simulink model "cdma_1"  (Simulink 7.8)
settings: Solver=ode45  StartTime=0.0  StopTime=10.0  RelTol=1e-3
undefined symbols (not defined in the file or in its folder): Fs, get, sided, Two
libraries: commrandsrc2 x10, commseqgen2 x10, commsink2 x3, dsparch4 x3, commutil2 x2, commdigbbndpm3 x2, dspsnks4 x2, commchan3 x1
settings Model: Creator=Administrator  LastModifiedBy=Administrator

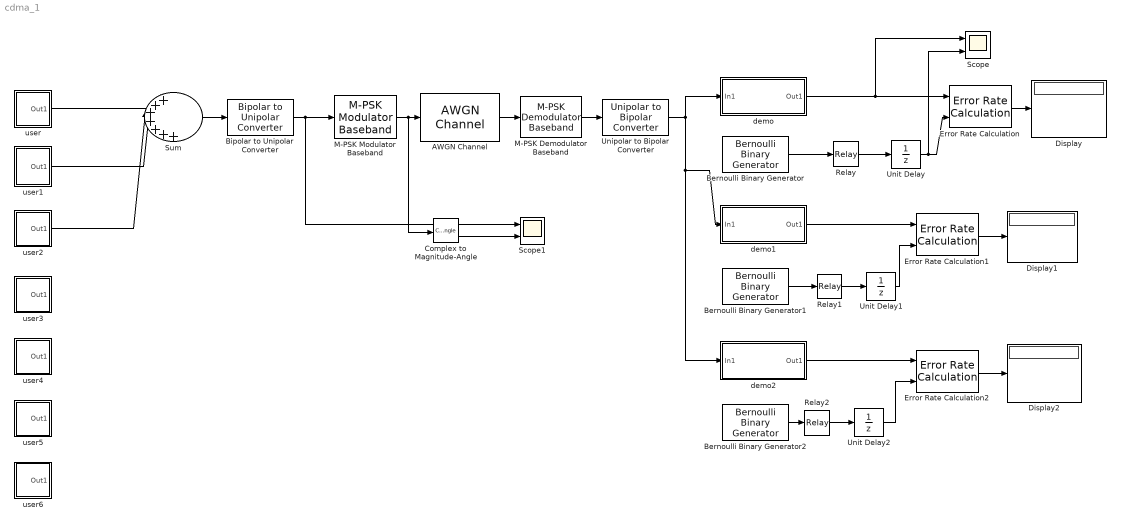
== system cdma_1 ==
  AWGN Channel : commchan3/AWGN Channel  InputProcessing=Columns as channels (frame based)  seed=1567  noiseMode="Signal to noise ratio  (SNR)"  EbNodB=10  EsNodB=10  SNRdB=10  bitsPerSym=1  Ps=1  Tsym=1  variance=1
  Bernoulli Binary Generator : commrandsrc2/Bernoulli Binary Generator  P=0.5  seed=67  Ts=6e-4  frameBased=off  sampPerFrame=1  orient=off  outDataType=double
  Bernoulli Binary Generator1 : commrandsrc2/Bernoulli Binary Generator  P=0.5  seed=71  Ts=6e-4  frameBased=off  sampPerFrame=1  orient=off  outDataType=double
  Bernoulli Binary Generator2 : commrandsrc2/Bernoulli Binary Generator  P=0.5  seed=87  Ts=6e-4  frameBased=off  sampPerFrame=1  orient=off  outDataType=double
  Bipolar to Unipolar Converter : commutil2/Bipolar to Unipolar Converter  M=4  polarity=Positive  dataType=Inherit via internal rule
  Complex to Magnitude-Angle : ComplexToMagnitudeAngle
  Display : Display
  Display1 : Display
  Display2 : Display
  Error Rate Calculation : commsink2/Error Rate Calculation  N=0  st_delay=0  cp_mode=Entire frame  subframe=[]  PMode=Port  WsName=ErrorVec  RsMode2=off  stop=off  numErr=100  maxBits=1e6
  Error Rate Calculation1 : commsink2/Error Rate Calculation  N=0  st_delay=0  cp_mode=Entire frame  subframe=[]  PMode=Port  WsName=ErrorVec  RsMode2=off  stop=off  numErr=100  maxBits=1e6
  Error Rate Calculation2 : commsink2/Error Rate Calculation  N=0  st_delay=0  cp_mode=Entire frame  subframe=[]  PMode=Port  WsName=ErrorVec  RsMode2=off  stop=off  numErr=100  maxBits=1e6
  M-PSK Demodulator Baseband : commdigbbndpm3/M-PSK Demodulator Baseband  M=4  Ph=pi/4  Dec=Gray  Mapping=[0:7]  OutType=Integer  DecType=Hard decision  VarSource=Dialog  Variance=1  outDtype1=Inherit via internal rule  outDtype2=Inherit via internal rule  derotateFactorWordLen=16
  M-PSK Modulator Baseband : commdigbbndpm3/M-PSK Modulator Baseband  M=4  InType=Integer  Enc=Gray  Mapping=[0:7]  Ph=pi/4  outDtype=double  outWordLen=16  outUDDataType=sfix(16)  outFracLenMode=Best precision  outFracLen=15
  Relay : Relay  OnSwitchValue=0.9  OffSwitchValue=0.1  OffOutputValue=-1
  Relay1 : Relay  OnSwitchValue=0.9  OffSwitchValue=0.1  OffOutputValue=-1
  Relay2 : Relay  OnSwitchValue=0.9  OffSwitchValue=0.1  OffOutputValue=-1
  Scope : Scope  NumInputPorts=2
      settings: YMin=-2~-2  YMax=2~2
  Scope1 : Scope  NumInputPorts=2
      settings: YMin=1~-2  YMax=6~4  SaveName=ScopeData2
  Sum : Sum  Inputs=|+++++++
  Unipolar to Bipolar Converter : commutil2/Unipolar to Bipolar Converter  M=4  polarity=Positive  dataType=Inherit via internal rule
  Unit Delay : UnitDelay  SampleTime=-1
  Unit Delay1 : UnitDelay  SampleTime=-1
  Unit Delay2 : UnitDelay  SampleTime=-1
  demo : Subsystem
  demo1 : Subsystem
  demo2 : Subsystem
  user : Subsystem
  user1 : Subsystem
  user2 : Subsystem
  user3 : Subsystem
  user4 : Subsystem
  user5 : Subsystem
  user6 : Subsystem
  wires:
  Error Rate Calculation/1 -> Display/1
  Bernoulli Binary Generator/1 -> Relay/1
  Relay/1 -> Unit Delay/1
  Relay1/1 -> Unit Delay1/1
  Bernoulli Binary Generator1/1 -> Relay1/1
  AWGN Channel/1 -> M-PSK Demodulator Baseband/1
  user1/1(Out1) -> Sum/2
  user/1(Out1) -> Sum/1
  M-PSK Modulator Baseband/1 -> AWGN Channel/1, Complex to Magnitude-Angle/1
  M-PSK Demodulator Baseband/1 -> Unipolar to Bipolar Converter/1
  Bipolar to Unipolar Converter/1 -> M-PSK Modulator Baseband/1, Scope1/1
  Unipolar to Bipolar Converter/1 -> demo/1(In1), demo1/1(In1), demo2/1(In1)
  demo1/1(Out1) -> Error Rate Calculation1/1
  Bernoulli Binary Generator2/1 -> Relay2/1
  Relay2/1 -> Unit Delay2/1
  Error Rate Calculation1/1 -> Display1/1
  demo2/1(Out1) -> Error Rate Calculation2/1
  Error Rate Calculation2/1 -> Display2/1
  Unit Delay1/1 -> Error Rate Calculation1/2
  Unit Delay/1 -> Error Rate Calculation/2, Scope/2
  demo/1(Out1) -> Error Rate Calculation/1, Scope/1
  Unit Delay2/1 -> Error Rate Calculation2/2
  Sum/1 -> Bipolar to Unipolar Converter/1
  Complex to Magnitude-Angle/2 -> Scope1/2
  user2/1(Out1) -> Sum/3

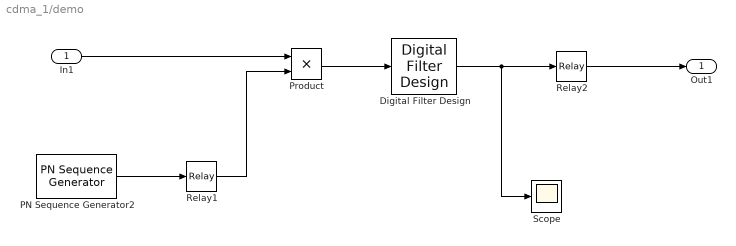
== system cdma_1/demo ==
  In1 : Inport
  Digital Filter Design : dsparch4/Digital Filter Design  mwdsp_browser_bugfix_var=off
  PN Sequence Generator2 : commseqgen2/PN Sequence Generator  poly=[1 0 0 0 0 1 1]  ini_sta=[0 0 0 0 0 1]  outBitMaskSource=Dialog parameter  shift=0  outVarSiz=off  maxOutSizeMode=Dialog parameter  maxOutSize=[10 1]  Ts=2e-5  frameBased=off  sampPerFrame=1  reset=off  bitPackedOutputs=off  outDataType=double  numPackedBits=8  bitPackDataSigned=off  bitPackedOutDType=double
  Product : Product  RndMeth=Zero
  Relay1 : Relay  OnSwitchValue=0.9  OffSwitchValue=0.1  OffOutputValue=-1
  Relay2 : Relay  OnSwitchValue=0  OffSwitchValue=0  OffOutputValue=-1  SampleTime=6e-4
  Scope : Scope
  Out1 : Outport
  wires:
  PN Sequence Generator2/1 -> Relay1/1
  Relay1/1 -> Product/2
  Relay2/1 -> Out1/1
  In1/1 -> Product/1
  Product/1 -> Digital Filter Design/1
  Digital Filter Design/1 -> Relay2/1, Scope/1

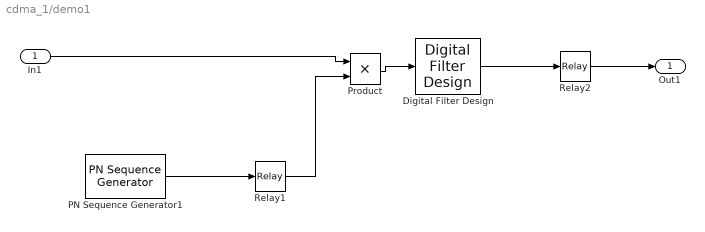
== system cdma_1/demo1 ==
  In1 : Inport
  Digital Filter Design : dsparch4/Digital Filter Design  mwdsp_browser_bugfix_var=off
  PN Sequence Generator1 : commseqgen2/PN Sequence Generator  poly=[1 0 0 0 0 1 1]  ini_sta=[1 0 0 0 0 0]  outBitMaskSource=Dialog parameter  shift=0  outVarSiz=off  maxOutSizeMode=Dialog parameter  maxOutSize=[10 1]  Ts=2e-5  frameBased=off  sampPerFrame=1  reset=off  bitPackedOutputs=off  outDataType=double  numPackedBits=8  bitPackDataSigned=off  bitPackedOutDType=double
  Product : Product  RndMeth=Zero
  Relay1 : Relay  OnSwitchValue=0.9  OffSwitchValue=0.1  OffOutputValue=-1
  Relay2 : Relay  OnSwitchValue=0  OffSwitchValue=0  OffOutputValue=-1  SampleTime=6e-4
  Out1 : Outport
  wires:
  Digital Filter Design/1 -> Relay2/1
  Relay1/1 -> Product/2
  Product/1 -> Digital Filter Design/1
  Relay2/1 -> Out1/1
  In1/1 -> Product/1
  PN Sequence Generator1/1 -> Relay1/1

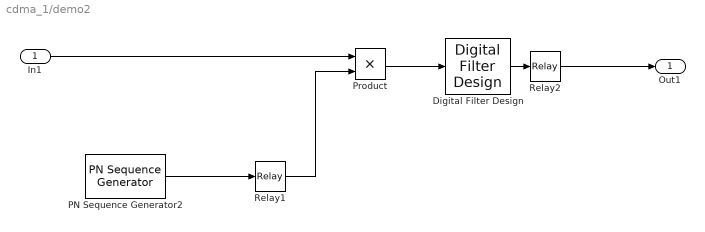
== system cdma_1/demo2 ==
  In1 : Inport
  Digital Filter Design : dsparch4/Digital Filter Design  mwdsp_browser_bugfix_var=off
  PN Sequence Generator2 : commseqgen2/PN Sequence Generator  poly=[1 0 0 0 0 1 1]  ini_sta=[1 1 0 0 0 0]  outBitMaskSource=Dialog parameter  shift=0  outVarSiz=off  maxOutSizeMode=Dialog parameter  maxOutSize=[10 1]  Ts=2e-5  frameBased=off  sampPerFrame=1  reset=off  bitPackedOutputs=off  outDataType=double  numPackedBits=8  bitPackDataSigned=off  bitPackedOutDType=double
  Product : Product  RndMeth=Zero
  Relay1 : Relay  OnSwitchValue=0.9  OffSwitchValue=0.1  OffOutputValue=-1
  Relay2 : Relay  OnSwitchValue=0  OffSwitchValue=0  OffOutputValue=-1  SampleTime=6e-4
  Out1 : Outport
  wires:
  Digital Filter Design/1 -> Relay2/1
  Relay1/1 -> Product/2
  Product/1 -> Digital Filter Design/1
  Relay2/1 -> Out1/1
  In1/1 -> Product/1
  PN Sequence Generator2/1 -> Relay1/1

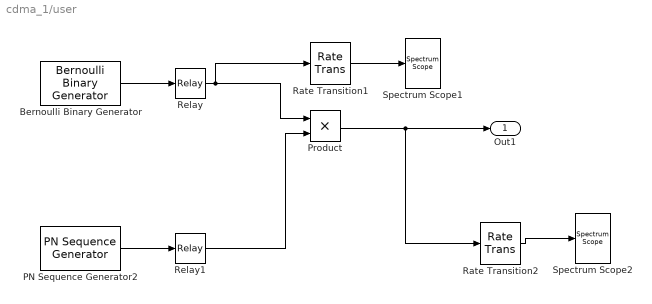
== system cdma_1/user ==
  Bernoulli Binary Generator : commrandsrc2/Bernoulli Binary Generator  P=0.5  seed=67  Ts=6e-4  frameBased=off  sampPerFrame=1  orient=off  outDataType=double
  PN Sequence Generator2 : commseqgen2/PN Sequence Generator  poly=[1 0 0 0 0 1 1]  ini_sta=[0 0 0 0 0 1]  outBitMaskSource=Dialog parameter  shift=0  outVarSiz=off  maxOutSizeMode=Dialog parameter  maxOutSize=[10 1]  Ts=2e-5  frameBased=off  sampPerFrame=1  reset=off  bitPackedOutputs=off  outDataType=double  numPackedBits=8  bitPackDataSigned=off  bitPackedOutDType=double
  Product : Product  RndMeth=Zero
  Rate Transition1 : RateTransition  OutPortSampleTime=1/10000
  Rate Transition2 : RateTransition  OutPortSampleTime=2/1000000
  Relay : Relay  OnSwitchValue=0.9  OffSwitchValue=0.1  OffOutputValue=-1
  Relay1 : Relay  OnSwitchValue=0.9  OffSwitchValue=0.1  OffOutputValue=-1
  Spectrum Scope1 : dspsnks4/Spectrum Scope  ScopeProperties=on  Domain=Frequency  HorizSpan=1  UseBuffer=on  BufferSize=2048  Overlap=0  TreatMby1Signals=One channel  inpFftLenInherit=off  FFTlength=128  numAvg=2  DisplayProperties=off  AxisGrid=on  Memory=off  FrameNumber=on  AxisLegend=off  AxisZoom=off  OpenScopeAtSimStart=on  OpenScopeImmediately=off  FigPos=get(0,'defaultfigureposition')  AxisProperties=off  XUnits=Hertz  XRange=Two-sided ((-Fs/2...Fs/2])  XDisplay=0  InheritXIncr=on  XIncr=1.0  XLabel=Samples  XLimit=Auto  YUnits=dBm  XMax=1  XMin=0  YLabel=Magnitude-squared, dB  LineProperties=off  wintypeSpecScope=Hann  RsSpecScope=50  betaSpecScope=5  winsampSpecScope=Periodic  XAxisParamsVer=6.9  isFrameUpgraded=on
      settings: YMin=-50  YMax=50
  Spectrum Scope2 : dspsnks4/Spectrum Scope  ScopeProperties=on  Domain=Frequency  HorizSpan=1  UseBuffer=on  BufferSize=1024  Overlap=0  TreatMby1Signals=One channel  inpFftLenInherit=off  FFTlength=128  numAvg=2  DisplayProperties=off  AxisGrid=on  Memory=off  FrameNumber=on  AxisLegend=off  AxisZoom=off  OpenScopeAtSimStart=on  OpenScopeImmediately=off  FigPos=get(0,'defaultfigureposition')  AxisProperties=off  XUnits=Hertz  XRange=Two-sided ((-Fs/2...Fs/2])  XDisplay=0  InheritXIncr=on  XIncr=1.0  XLabel=Samples  XLimit=Auto  YUnits=dBm  XMax=1  XMin=0  YLabel=Magnitude-squared, dB  LineProperties=off  wintypeSpecScope=Hann  RsSpecScope=50  betaSpecScope=5  winsampSpecScope=Periodic  XAxisParamsVer=6.9  isFrameUpgraded=on
      settings: YMin=-50  YMax=50
  Out1 : Outport
  wires:
  Bernoulli Binary Generator/1 -> Relay/1
  PN Sequence Generator2/1 -> Relay1/1
  Relay/1 -> Rate Transition1/1, Product/1
  Relay1/1 -> Product/2
  Product/1 -> Out1/1, Rate Transition2/1
  Rate Transition1/1 -> Spectrum Scope1/1
  Rate Transition2/1 -> Spectrum Scope2/1

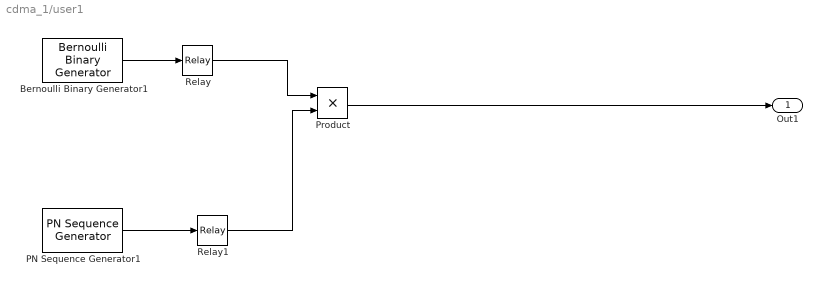
== system cdma_1/user1 ==
  Bernoulli Binary Generator1 : commrandsrc2/Bernoulli Binary Generator  P=0.5  seed=71  Ts=6e-4  frameBased=off  sampPerFrame=1  orient=off  outDataType=double
  PN Sequence Generator1 : commseqgen2/PN Sequence Generator  poly=[1 0 0 0 0 1 1]  ini_sta=[1 0 0 0 0 0]  outBitMaskSource=Dialog parameter  shift=0  outVarSiz=off  maxOutSizeMode=Dialog parameter  maxOutSize=[10 1]  Ts=2e-5  frameBased=off  sampPerFrame=1  reset=off  bitPackedOutputs=off  outDataType=double  numPackedBits=8  bitPackDataSigned=off  bitPackedOutDType=double
  Product : Product  RndMeth=Zero
  Relay : Relay  OnSwitchValue=0.9  OffSwitchValue=0.1  OffOutputValue=-1
  Relay1 : Relay  OnSwitchValue=0.9  OffSwitchValue=0.1  OffOutputValue=-1
  Out1 : Outport
  wires:
  Bernoulli Binary Generator1/1 -> Relay/1
  Relay/1 -> Product/1
  Relay1/1 -> Product/2
  PN Sequence Generator1/1 -> Relay1/1
  Product/1 -> Out1/1

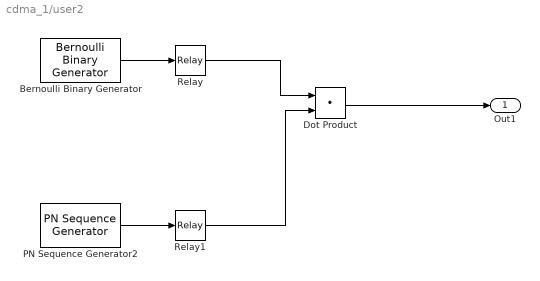
== system cdma_1/user2 ==
  Bernoulli Binary Generator : commrandsrc2/Bernoulli Binary Generator  P=0.5  seed=87  Ts=6e-4  frameBased=off  sampPerFrame=1  orient=off  outDataType=double
  Dot Product : DotProduct  InputSameDT=on  OutDataTypeStr=Inherit: Inherit via internal rule
  PN Sequence Generator2 : commseqgen2/PN Sequence Generator  poly=[1 0 0 0 0 1 1]  ini_sta=[1 1 0 0 0 0]  outBitMaskSource=Dialog parameter  shift=0  outVarSiz=off  maxOutSizeMode=Dialog parameter  maxOutSize=[10 1]  Ts=2e-5  frameBased=off  sampPerFrame=1  reset=off  bitPackedOutputs=off  outDataType=double  numPackedBits=8  bitPackDataSigned=off  bitPackedOutDType=double
  Relay : Relay  OnSwitchValue=0.9  OffSwitchValue=0.1  OffOutputValue=-1
  Relay1 : Relay  OnSwitchValue=0.9  OffSwitchValue=0.1  OffOutputValue=-1
  Out1 : Outport
  wires:
  Bernoulli Binary Generator/1 -> Relay/1
  PN Sequence Generator2/1 -> Relay1/1
  Relay/1 -> Dot Product/1
  Relay1/1 -> Dot Product/2
  Dot Product/1 -> Out1/1

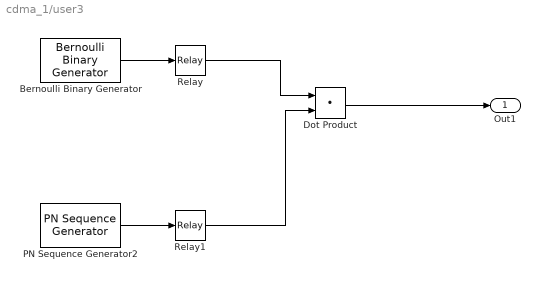
== system cdma_1/user3 ==
  Bernoulli Binary Generator : commrandsrc2/Bernoulli Binary Generator  P=0.5  seed=88  Ts=6e-4  frameBased=off  sampPerFrame=1  orient=off  outDataType=double
  Dot Product : DotProduct  InputSameDT=on  OutDataTypeStr=Inherit: Inherit via internal rule
  PN Sequence Generator2 : commseqgen2/PN Sequence Generator  poly=[1 0 0 0 0 1 1]  ini_sta=[1 1 1 0 0 0]  outBitMaskSource=Dialog parameter  shift=0  outVarSiz=off  maxOutSizeMode=Dialog parameter  maxOutSize=[10 1]  Ts=2e-5  frameBased=off  sampPerFrame=1  reset=off  bitPackedOutputs=off  outDataType=double  numPackedBits=8  bitPackDataSigned=off  bitPackedOutDType=double
  Relay : Relay  OnSwitchValue=0.9  OffSwitchValue=0.1  OffOutputValue=-1
  Relay1 : Relay  OnSwitchValue=0.9  OffSwitchValue=0.1  OffOutputValue=-1
  Out1 : Outport
  wires:
  Bernoulli Binary Generator/1 -> Relay/1
  PN Sequence Generator2/1 -> Relay1/1
  Relay/1 -> Dot Product/1
  Relay1/1 -> Dot Product/2
  Dot Product/1 -> Out1/1

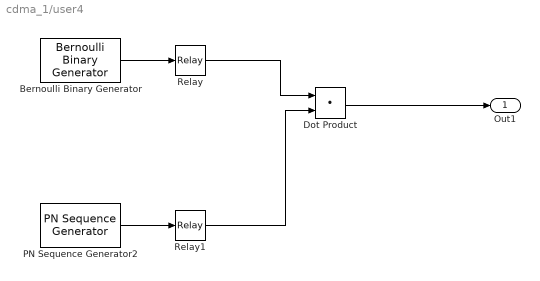
== system cdma_1/user4 ==
  Bernoulli Binary Generator : commrandsrc2/Bernoulli Binary Generator  P=0.5  seed=89  Ts=6e-4  frameBased=off  sampPerFrame=1  orient=off  outDataType=double
  Dot Product : DotProduct  InputSameDT=on  OutDataTypeStr=Inherit: Inherit via internal rule
  PN Sequence Generator2 : commseqgen2/PN Sequence Generator  poly=[1 0 0 0 0 1 1]  ini_sta=[1 1 1 1 0 0]  outBitMaskSource=Dialog parameter  shift=0  outVarSiz=off  maxOutSizeMode=Dialog parameter  maxOutSize=[10 1]  Ts=2e-5  frameBased=off  sampPerFrame=1  reset=off  bitPackedOutputs=off  outDataType=double  numPackedBits=8  bitPackDataSigned=off  bitPackedOutDType=double
  Relay : Relay  OnSwitchValue=0.9  OffSwitchValue=0.1  OffOutputValue=-1
  Relay1 : Relay  OnSwitchValue=0.9  OffSwitchValue=0.1  OffOutputValue=-1
  Out1 : Outport
  wires:
  Bernoulli Binary Generator/1 -> Relay/1
  PN Sequence Generator2/1 -> Relay1/1
  Relay/1 -> Dot Product/1
  Relay1/1 -> Dot Product/2
  Dot Product/1 -> Out1/1

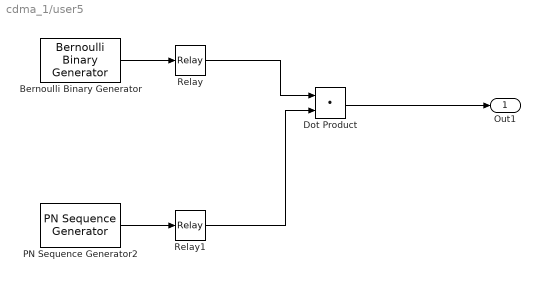
== system cdma_1/user5 ==
  Bernoulli Binary Generator : commrandsrc2/Bernoulli Binary Generator  P=0.5  seed=90  Ts=6e-4  frameBased=off  sampPerFrame=1  orient=off  outDataType=double
  Dot Product : DotProduct  InputSameDT=on  OutDataTypeStr=Inherit: Inherit via internal rule
  PN Sequence Generator2 : commseqgen2/PN Sequence Generator  poly=[1 0 0 0 0 1 1]  ini_sta=[1 1 1 1 1 0]  outBitMaskSource=Dialog parameter  shift=0  outVarSiz=off  maxOutSizeMode=Dialog parameter  maxOutSize=[10 1]  Ts=2e-5  frameBased=off  sampPerFrame=1  reset=off  bitPackedOutputs=off  outDataType=double  numPackedBits=8  bitPackDataSigned=off  bitPackedOutDType=double
  Relay : Relay  OnSwitchValue=0.9  OffSwitchValue=0.1  OffOutputValue=-1
  Relay1 : Relay  OnSwitchValue=0.9  OffSwitchValue=0.1  OffOutputValue=-1
  Out1 : Outport
  wires:
  Bernoulli Binary Generator/1 -> Relay/1
  PN Sequence Generator2/1 -> Relay1/1
  Relay/1 -> Dot Product/1
  Relay1/1 -> Dot Product/2
  Dot Product/1 -> Out1/1

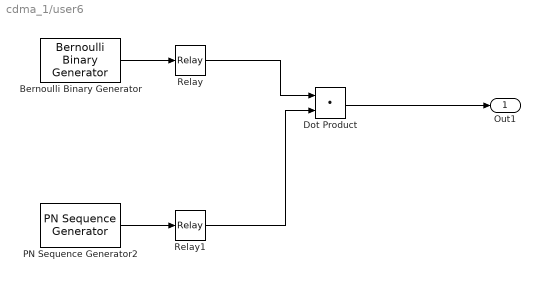
== system cdma_1/user6 ==
  Bernoulli Binary Generator : commrandsrc2/Bernoulli Binary Generator  P=0.5  seed=100  Ts=6e-4  frameBased=off  sampPerFrame=1  orient=off  outDataType=double
  Dot Product : DotProduct  InputSameDT=on  OutDataTypeStr=Inherit: Inherit via internal rule
  PN Sequence Generator2 : commseqgen2/PN Sequence Generator  poly=[1 0 0 0 0 1 1]  ini_sta=[1 1 1 1 1 1]  outBitMaskSource=Dialog parameter  shift=0  outVarSiz=off  maxOutSizeMode=Dialog parameter  maxOutSize=[10 1]  Ts=2e-5  frameBased=off  sampPerFrame=1  reset=off  bitPackedOutputs=off  outDataType=double  numPackedBits=8  bitPackDataSigned=off  bitPackedOutDType=double
  Relay : Relay  OnSwitchValue=0.9  OffSwitchValue=0.1  OffOutputValue=-1
  Relay1 : Relay  OnSwitchValue=0.9  OffSwitchValue=0.1  OffOutputValue=-1
  Out1 : Outport
  wires:
  Bernoulli Binary Generator/1 -> Relay/1
  PN Sequence Generator2/1 -> Relay1/1
  Relay/1 -> Dot Product/1
  Relay1/1 -> Dot Product/2
  Dot Product/1 -> Out1/1
